simulink model "EV_Battery_Pack_modelling"  (R2023b)
settings: Solver=VariableStepAuto  StartTime=0.0  StopTime=2472  RelTol=1e-3
undefined symbols (not defined in the file or in its folder): Ion, Lithium
libraries: spsBatteryLib x12, spsControlledCurrentSourceLib x1, autolibshared x1, spsVoltageMeasurementLib x1, sps_lib x1
settings Model: SimulationMode=rapid-accelerator  Creator=varda  LastModifiedBy=varda
settings SolverCC: ZeroCrossControl=EnableAll  ZeroCrossAlgorithm=Adaptive
settings DebuggingCC: IgnoredZcDiagnostic=none

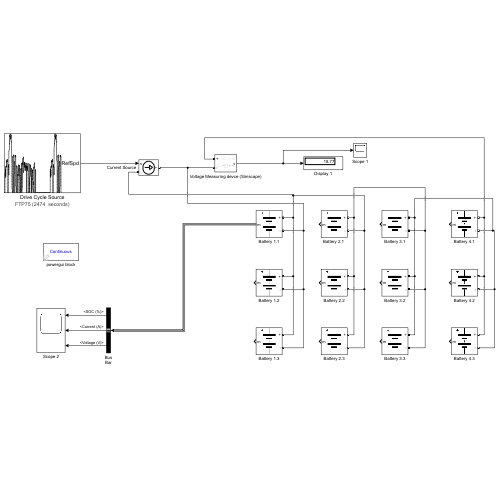
[thumbnail: Simulink's stored preview of the top-level diagram]
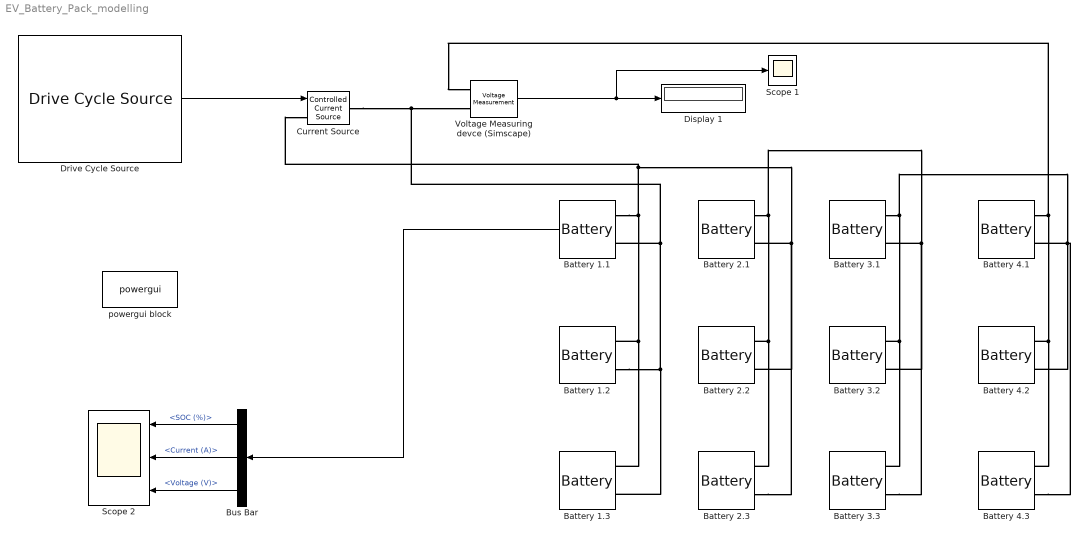
== system EV_Battery_Pack_modelling ==
  Battery 1.1 : spsBatteryLib/Battery  BatType=Lithium-Ion  ShowTempParam=off  ThermalPreset=no  ShowAgeParam=off  NomV=4.2  NomQ=1.3  SOC=100  Batt_Tr=30  PresetModel=on  MaxQ=1.3  MinV=3.15  FullV=4.8887  Dis_rate=0.56522  R=0.032308  Normal_OP=1.1757  expZone="[4.5376     0.06387]"  current=[6.5 13 32.5]  Units=Time  Tci=20  NomT=20  T2=-30  MaxQ2=4.8  FullV2=7.1  Normal_OP2=5.655  expZone2="[6.58           1]"  Rca=0.6  ti=2000  Dp=0  Neq0=0  Tsim=1e6  Ta1=25  Qeol=5.4*0.9  Reol=0.013333*1.2  Char_age=[2.3478, 3]  Dis_age=[2.3478, 10]  N1=1500  N2=10500  N3=1000  N4=1400  Ta2=45  N5=950
  Battery 1.2 : spsBatteryLib/Battery  BatType=Lithium-Ion  ShowTempParam=off  ThermalPreset=no  ShowAgeParam=off  NomV=4.2  NomQ=1.3  SOC=100  Batt_Tr=30  PresetModel=on  MaxQ=1.3  MinV=3.15  FullV=4.8887  Dis_rate=0.56522  R=0.032308  Normal_OP=1.1757  expZone="[4.5376     0.06387]"  current=[6.5 13 32.5]  Units=Time  Tci=20  NomT=20  T2=-30  MaxQ2=4.8  FullV2=7.1  Normal_OP2=5.655  expZone2="[6.58           1]"  Rca=0.6  ti=2000  Dp=0  Neq0=0  Tsim=1e6  Ta1=25  Qeol=5.4*0.9  Reol=0.013333*1.2  Char_age=[2.3478, 3]  Dis_age=[2.3478, 10]  N1=1500  N2=10500  N3=1000  N4=1400  Ta2=45  N5=950
  Battery 1.3 : spsBatteryLib/Battery  BatType=Lithium-Ion  ShowTempParam=off  ThermalPreset=no  ShowAgeParam=off  NomV=4.2  NomQ=1.3  SOC=100  Batt_Tr=30  PresetModel=on  MaxQ=1.3  MinV=3.15  FullV=4.8887  Dis_rate=0.56522  R=0.032308  Normal_OP=1.1757  expZone="[4.5376     0.06387]"  current=[6.5 13 32.5]  Units=Time  Tci=20  NomT=20  T2=-30  MaxQ2=4.8  FullV2=7.1  Normal_OP2=5.655  expZone2="[6.58           1]"  Rca=0.6  ti=2000  Dp=0  Neq0=0  Tsim=1e6  Ta1=25  Qeol=5.4*0.9  Reol=0.013333*1.2  Char_age=[2.3478, 3]  Dis_age=[2.3478, 10]  N1=1500  N2=10500  N3=1000  N4=1400  Ta2=45  N5=950
  "Battery 2.1 " : spsBatteryLib/Battery  BatType=Lithium-Ion  ShowTempParam=off  ThermalPreset=no  ShowAgeParam=off  NomV=4.2  NomQ=1.3  SOC=100  Batt_Tr=30  PresetModel=on  MaxQ=1.3  MinV=3.15  FullV=4.8887  Dis_rate=0.56522  R=0.032308  Normal_OP=1.1757  expZone="[4.5376     0.06387]"  current=[6.5 13 32.5]  Units=Time  Tci=20  NomT=20  T2=-30  MaxQ2=4.8  FullV2=7.1  Normal_OP2=5.655  expZone2="[6.58           1]"  Rca=0.6  ti=2000  Dp=0  Neq0=0  Tsim=1e6  Ta1=25  Qeol=5.4*0.9  Reol=0.013333*1.2  Char_age=[2.3478, 3]  Dis_age=[2.3478, 10]  N1=1500  N2=10500  N3=1000  N4=1400  Ta2=45  N5=950
  Battery 2.2 : spsBatteryLib/Battery  BatType=Lithium-Ion  ShowTempParam=off  ThermalPreset=no  ShowAgeParam=off  NomV=4.2  NomQ=1.3  SOC=100  Batt_Tr=30  PresetModel=on  MaxQ=1.3  MinV=3.15  FullV=4.8887  Dis_rate=0.56522  R=0.032308  Normal_OP=1.1757  expZone="[4.5376     0.06387]"  current=[6.5 13 32.5]  Units=Time  Tci=20  NomT=20  T2=-30  MaxQ2=4.8  FullV2=7.1  Normal_OP2=5.655  expZone2="[6.58           1]"  Rca=0.6  ti=2000  Dp=0  Neq0=0  Tsim=1e6  Ta1=25  Qeol=5.4*0.9  Reol=0.013333*1.2  Char_age=[2.3478, 3]  Dis_age=[2.3478, 10]  N1=1500  N2=10500  N3=1000  N4=1400  Ta2=45  N5=950
  Battery 2.3 : spsBatteryLib/Battery  BatType=Lithium-Ion  ShowTempParam=off  ThermalPreset=no  ShowAgeParam=off  NomV=4.2  NomQ=1.3  SOC=100  Batt_Tr=30  PresetModel=on  MaxQ=1.3  MinV=3.15  FullV=4.8887  Dis_rate=0.56522  R=0.032308  Normal_OP=1.1757  expZone="[4.5376     0.06387]"  current=[6.5 13 32.5]  Units=Time  Tci=20  NomT=20  T2=-30  MaxQ2=4.8  FullV2=7.1  Normal_OP2=5.655  expZone2="[6.58           1]"  Rca=0.6  ti=2000  Dp=0  Neq0=0  Tsim=1e6  Ta1=25  Qeol=5.4*0.9  Reol=0.013333*1.2  Char_age=[2.3478, 3]  Dis_age=[2.3478, 10]  N1=1500  N2=10500  N3=1000  N4=1400  Ta2=45  N5=950
  Battery 3.1 : spsBatteryLib/Battery  BatType=Lithium-Ion  ShowTempParam=off  ThermalPreset=no  ShowAgeParam=off  NomV=4.2  NomQ=1.3  SOC=100  Batt_Tr=30  PresetModel=on  MaxQ=1.3  MinV=3.15  FullV=4.8887  Dis_rate=0.56522  R=0.032308  Normal_OP=1.1757  expZone="[4.5376     0.06387]"  current=[6.5 13 32.5]  Units=Time  Tci=20  NomT=20  T2=-30  MaxQ2=4.8  FullV2=7.1  Normal_OP2=5.655  expZone2="[6.58           1]"  Rca=0.6  ti=2000  Dp=0  Neq0=0  Tsim=1e6  Ta1=25  Qeol=5.4*0.9  Reol=0.013333*1.2  Char_age=[2.3478, 3]  Dis_age=[2.3478, 10]  N1=1500  N2=10500  N3=1000  N4=1400  Ta2=45  N5=950
  Battery 3.2 : spsBatteryLib/Battery  BatType=Lithium-Ion  ShowTempParam=off  ThermalPreset=no  ShowAgeParam=off  NomV=4.2  NomQ=1.3  SOC=100  Batt_Tr=30  PresetModel=on  MaxQ=1.3  MinV=3.15  FullV=4.8887  Dis_rate=0.56522  R=0.032308  Normal_OP=1.1757  expZone="[4.5376     0.06387]"  current=[6.5 13 32.5]  Units=Time  Tci=20  NomT=20  T2=-30  MaxQ2=4.8  FullV2=7.1  Normal_OP2=5.655  expZone2="[6.58           1]"  Rca=0.6  ti=2000  Dp=0  Neq0=0  Tsim=1e6  Ta1=25  Qeol=5.4*0.9  Reol=0.013333*1.2  Char_age=[2.3478, 3]  Dis_age=[2.3478, 10]  N1=1500  N2=10500  N3=1000  N4=1400  Ta2=45  N5=950
  Battery 3.3 : spsBatteryLib/Battery  BatType=Lithium-Ion  ShowTempParam=off  ThermalPreset=no  ShowAgeParam=off  NomV=4.2  NomQ=1.3  SOC=100  Batt_Tr=30  PresetModel=on  MaxQ=1.3  MinV=3.15  FullV=4.8887  Dis_rate=0.56522  R=0.032308  Normal_OP=1.1757  expZone="[4.5376     0.06387]"  current=[6.5 13 32.5]  Units=Time  Tci=20  NomT=20  T2=-30  MaxQ2=4.8  FullV2=7.1  Normal_OP2=5.655  expZone2="[6.58           1]"  Rca=0.6  ti=2000  Dp=0  Neq0=0  Tsim=1e6  Ta1=25  Qeol=5.4*0.9  Reol=0.013333*1.2  Char_age=[2.3478, 3]  Dis_age=[2.3478, 10]  N1=1500  N2=10500  N3=1000  N4=1400  Ta2=45  N5=950
  Battery 4.1 : spsBatteryLib/Battery  BatType=Lithium-Ion  ShowTempParam=off  ThermalPreset=no  ShowAgeParam=off  NomV=4.2  NomQ=1.3  SOC=100  Batt_Tr=30  PresetModel=on  MaxQ=1.3  MinV=3.15  FullV=4.8887  Dis_rate=0.56522  R=0.032308  Normal_OP=1.1757  expZone="[4.5376     0.06387]"  current=[6.5 13 32.5]  Units=Time  Tci=20  NomT=20  T2=-30  MaxQ2=4.8  FullV2=7.1  Normal_OP2=5.655  expZone2="[6.58           1]"  Rca=0.6  ti=2000  Dp=0  Neq0=0  Tsim=1e6  Ta1=25  Qeol=5.4*0.9  Reol=0.013333*1.2  Char_age=[2.3478, 3]  Dis_age=[2.3478, 10]  N1=1500  N2=10500  N3=1000  N4=1400  Ta2=45  N5=950
  Battery 4.2 : spsBatteryLib/Battery  BatType=Lithium-Ion  ShowTempParam=off  ThermalPreset=no  ShowAgeParam=off  NomV=4.2  NomQ=1.3  SOC=100  Batt_Tr=30  PresetModel=on  MaxQ=1.3  MinV=3.15  FullV=4.8887  Dis_rate=0.56522  R=0.032308  Normal_OP=1.1757  expZone="[4.5376     0.06387]"  current=[6.5 13 32.5]  Units=Time  Tci=20  NomT=20  T2=-30  MaxQ2=4.8  FullV2=7.1  Normal_OP2=5.655  expZone2="[6.58           1]"  Rca=0.6  ti=2000  Dp=0  Neq0=0  Tsim=1e6  Ta1=25  Qeol=5.4*0.9  Reol=0.013333*1.2  Char_age=[2.3478, 3]  Dis_age=[2.3478, 10]  N1=1500  N2=10500  N3=1000  N4=1400  Ta2=45  N5=950
  Battery 4.3 : spsBatteryLib/Battery  BatType=Lithium-Ion  ShowTempParam=off  ThermalPreset=no  ShowAgeParam=off  NomV=4.2  NomQ=1.3  SOC=100  Batt_Tr=30  PresetModel=on  MaxQ=1.3  MinV=3.15  FullV=4.8887  Dis_rate=0.56522  R=0.032308  Normal_OP=1.1757  expZone="[4.5376     0.06387]"  current=[6.5 13 32.5]  Units=Time  Tci=20  NomT=20  T2=-30  MaxQ2=4.8  FullV2=7.1  Normal_OP2=5.655  expZone2="[6.58           1]"  Rca=0.6  ti=2000  Dp=0  Neq0=0  Tsim=1e6  Ta1=25  Qeol=5.4*0.9  Reol=0.013333*1.2  Char_age=[2.3478, 3]  Dis_age=[2.3478, 10]  N1=1500  N2=10500  N3=1000  N4=1400  Ta2=45  N5=950
  Bus Bar : BusSelector  OutputSignals=SOC (%),Current (A),Voltage (V)
  Current Source : spsControlledCurrentSourceLib/Controlled Current Source  Initialize=on  Source_Type=AC  Amplitude=0  Phase=0  Frequency=0  Measurements=None
  Display 1 : Display
  Drive Cycle Source : autolibshared/Drive Cycle Source  cycleVar=FTP75  fileVar=cycleFTP75.mat  tfinal="2474  seconds"  cycleRepeat=off  outAccPort=off  outGearPort=off  gearList=No gear data  t_wot1=5  xdot_woto=0  xdot_wot1=30  t_wot2=20  xdot_wot2=0  t_wotend=30  srcUnit=m/s  outUnit=m/s  srcAccUnit=m/s/s  outAccUnit=m/s^2  dt=0  aMode=1  faultOption=off  velBnd=2  velBndUnit=mph  inUnit=m/s  timeBnd=1  failOption=off  stopSim=off  maxFaultCnt=10  maxFaultTime=2  maxTotFaultTime=15  traceOption=off  dtTrace=1  traceWindow=10  lastDCname=FTP75  lastOutUnit=mph  lastDT=0  lastTB=1  lastSB=2  forceCalcBound=off
  Scope 1 : Scope
  Scope 2 : Scope  NumInputPorts=3
  Voltage Measuring devce (Simscape) : spsVoltageMeasurementLib/Voltage Measurement  PhasorSimulation=off  OutputType=Complex  PSBequivalent=0
  powergui block : sps_lib/powergui  Priority=1  SimulationMode=Continuous  SampleTime=50e-6  frequency=60  Iterations=50  frequencyindice=0  Pbase=100e6  ErrMax=1e-4  UnitsV=kV  UnitsW=MW  buscounter=0  FunctionMessages=off  echomessages=off  EnableUseOfTLC=off  CurrentSourceSwitches=off  DisableSnubberDevices=off  DisableRonSwitches=off  DisableVfSwitches=off  DisplayEquations=off  AutomaticDiscreteSolvers=off  SolverType=Tustin/Backward Euler (TBE)  Interpol=off  ExternalGateDelay=off  methode=off  Ts=100  x0status=blocks  SPID=on  SwTol=0  HookPort=off  NonlinearTolerance=1e-4  nMaxIteration=100  ContinueOnMaxIteration=off  RestoreLinks=warning  ResistiveCurrentMeasurement=off  Frange=[0:2:500]  Ylog=off  Xlog=on  ShowGrid=off  save=off  variable=ZData  structure=0  ZoomFFT=off  StartTime=0.0  cycles=1  DisplayStyle=1  fundamental=60  FreqAxis=off  MaxFrequency=1000  frequencyindicesteady=1  RmsSteady=1  display=off
  wires:
  Voltage Measuring devce (Simscape)/1 -> Scope 1/1, Display 1/1
  Drive Cycle Source/1 -> Current Source/1
  Battery 1.1/1 -> Bus Bar/1
  Bus Bar/1 -> Scope 2/1  "<SOC (%)>"
  Bus Bar/2 -> Scope 2/2  "<Current (A)>"
  Bus Bar/3 -> Scope 2/3  "<Voltage (V)>"
  connections:
  Battery 1.2/LConn2 -- Battery 1.3/LConn2 -- Voltage Measuring devce (Simscape)/LConn2 -- Current Source/RConn1 -- Battery 1.1/LConn2
  Battery 1.1/LConn1 -- Battery 1.2/LConn1 -- Battery 1.3/LConn1 -- Battery 2.3/LConn2 -- Battery 2.2/LConn2 -- "Battery 2.1 "/LConn2 -- Current Source/LConn1
  "Battery 2.1 "/LConn1 -- Battery 3.1/LConn2 -- Battery 3.3/LConn2 -- Battery 3.2/LConn2 -- Battery 2.3/LConn1 -- Battery 2.2/LConn1
  Battery 4.1/LConn1 -- Battery 4.3/LConn1 -- Battery 4.2/LConn1 -- Voltage Measuring devce (Simscape)/LConn1
  Battery 3.1/LConn1 -- Battery 3.3/LConn1 -- Battery 3.2/LConn1 -- Battery 4.1/LConn2 -- Battery 4.2/LConn2 -- Battery 4.3/LConn2
